simulink model "Highpass_filter"  (R2020b)
settings: Solver=VariableStepAuto  StartTime=0.0  StopTime=10.0  RelTol=1e-3
values from neighbouring files (symbols this model uses):
  h1 = 0.1548    [values.m]
  h2 = -0.5792    [values.m]
settings Model: Creator=Abhinav dixit  LastModifiedBy=Abhinav dixit

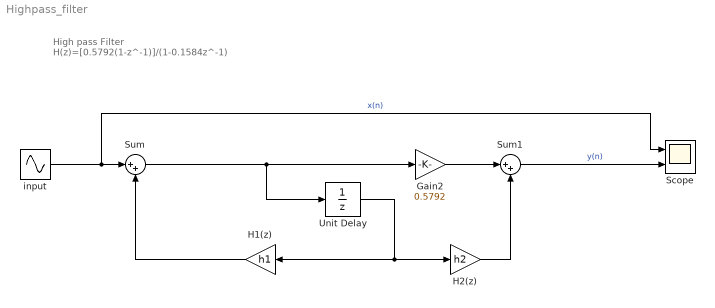
== system Highpass_filter ==
  note: High pass Filter
      | H(z)=[0.5792(1-z^-1)]/(1-0.1584z^-1)
  Gain2 : Gain  Gain=0.5792
  H1(z) : Gain  Gain=h1
  H2(z) : Gain  Gain=h2
  Scope : Scope  NumInputPorts=2
  Sum : Sum  Inputs=|++
  Sum1 : Sum  Inputs=|++
  Unit Delay : UnitDelay  SampleTime=-1  HasFrameUpgradeWarning=on
  input : Sin  Frequency=10000  SampleTime=0
  wires:
  input/1 -> Scope/1, Sum/1  "x(n)"
  Sum/1 -> Gain2/1, Unit Delay/1
  Unit Delay/1 -> H2(z)/1, H1(z)/1
  H1(z)/1 -> Sum/2
  H2(z)/1 -> Sum1/2
  Sum1/1 -> Scope/2  "y(n)"
  Gain2/1 -> Sum1/1
